simulink model "model_lqr_1D"  (R2016b)
settings: Solver=FixedStepAuto  StartTime=0.0  StopTime=15  FixedStep=0.001  RelTol=1e-3  EnableMultiTasking=on
InitFcn:
  | initCallback_model1D
values from neighbouring files (symbols this model uses):
  C_phi = 6.2e-3    (= 0.0062)    [initCallback_model1D.m]
  C_psi = 3.1176e-5    (= 3.1176e-05)    [initCallback_model1D.m]
  g = 9.81    [initCallback_model1D.m]
  I_GO = I_KO + I_RM + m_R * l_AB^2    (= 0.00355187)    [initCallback_model1D.m]
  I_RM = 1.1683e-4    (= 0.00011683)    [initCallback_model1D.m]
  l_AB = 0.084    [initCallback_model1D.m]
  l_AC = 0.087    [initCallback_model1D.m]
  m_K = 0.221    [initCallback_model1D.m]
  m_R = 0.09    [initCallback_model1D.m]
  phi_0 = degtorad(3)    [initCallback_model1D.m]
  phi__d_0 = 0    [initCallback_model1D.m]
  psi_0 = 0    [initCallback_model1D.m]
  psi__d_0 = 0    [initCallback_model1D.m]
  T_M_e = 5.5e-4    (= 0.00055)    [initCallback_model1D.m]
  T_M_m = 12.4e-3    (= 0.0124)    [initCallback_model1D.m]
settings Model: Creator=ich  LastModifiedBy=ich
settings SolverCC: AutoInsertRateTranBlk=on
settings OptimizationCC: LifeSpan=inf
settings DebuggingCC: SFUnexpectedBacktrackingDiag=warning  SFNoUnconditionalDefaultTransitionDiag=warning  SFExecutionAtInitializationDiag=none
settings GRTTargetCC: TargetLangStandard=C89/C90 (ANSI)  GeneratePreprocessorConditionals=Disable all
settings ConfigComp: CovMetricSettings=dw  CovHtmlReporting=on  CovSaveCumulativeToWorkspaceVar=on  CovSaveSingleToWorkspaceVar=on  CovExternalEMLEnable=off

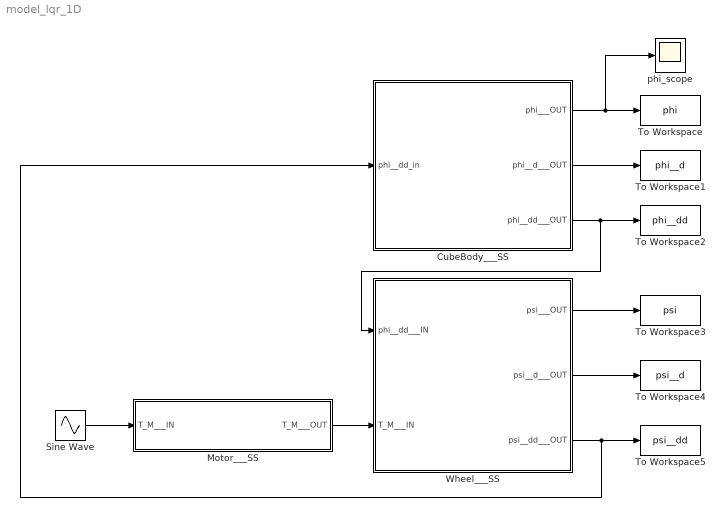
== system model_lqr_1D ==
  CubeBody___SS : Subsystem
  Motor___SS : Subsystem
  Sine Wave : Sin  Amplitude=0.05  SampleTime=0
  To Workspace : ToWorkspace  VariableName=phi  SaveFormat=Timeseries  SampleTime=-1
  To Workspace1 : ToWorkspace  VariableName=phi__d  SaveFormat=Timeseries  SampleTime=-1
  To Workspace2 : ToWorkspace  VariableName=phi__dd  SaveFormat=Timeseries  SampleTime=-1
  To Workspace3 : ToWorkspace  VariableName=psi  SaveFormat=Timeseries  SampleTime=-1
  To Workspace4 : ToWorkspace  VariableName=psi__d  SaveFormat=Timeseries  SampleTime=-1
  To Workspace5 : ToWorkspace  VariableName=psi__dd  SaveFormat=Timeseries  SampleTime=-1
  Wheel___SS : Subsystem
  phi_scope : Scope
  wires:
  Motor___SS/1(T_M___OUT) -> Wheel___SS/2(T_M___IN)
  CubeBody___SS/3(phi__dd___OUT) -> Wheel___SS/1(phi__dd___IN), To Workspace2/1
  Wheel___SS/3(psi__dd___OUT) -> To Workspace5/1, CubeBody___SS/1(phi__dd_in)
  CubeBody___SS/1(phi___OUT) -> phi_scope/1, To Workspace/1
  CubeBody___SS/2(phi__d___OUT) -> To Workspace1/1
  Wheel___SS/1(psi___OUT) -> To Workspace3/1
  Wheel___SS/2(psi__d___OUT) -> To Workspace4/1
  Sine Wave/1 -> Motor___SS/1(T_M___IN)

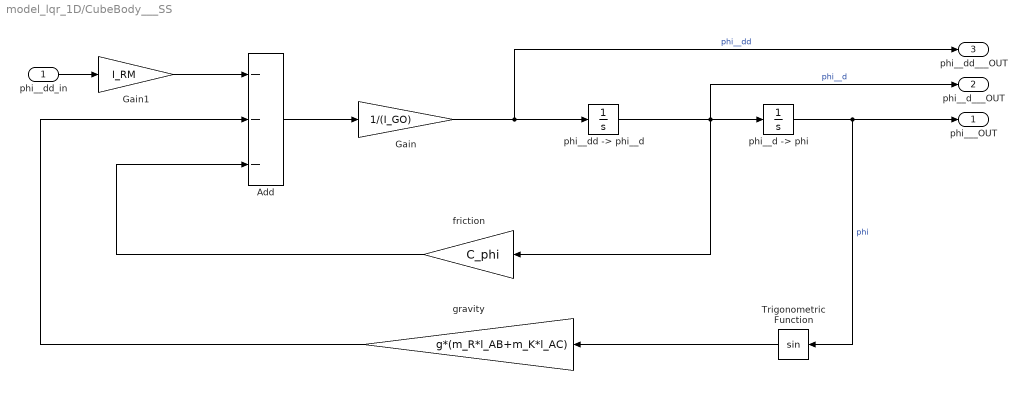
== system model_lqr_1D/CubeBody___SS ==
  phi__dd_in : Inport
  Add : Sum  Inputs=---
  Gain : Gain  Gain=1/(I_GO)
  Gain1 : Gain  Gain=I_RM
  Trigonometric Function : Trigonometry
  friction : Gain  Gain=C_phi
  gravity : Gain  Gain=g*(m_R*l_AB+m_K*l_AC)
  "phi__d -> phi" : Integrator  InitialCondition=phi_0
  "phi__dd -> phi__d" : Integrator  InitialCondition=phi__d_0
  phi___OUT : Outport
  phi__d___OUT : Outport  Port=2
  phi__dd___OUT : Outport  Port=3
  wires:
  "phi__d -> phi"/1 -> Trigonometric Function/1, phi___OUT/1  "phi"
  "phi__dd -> phi__d"/1 -> friction/1, phi__d___OUT/1, "phi__d -> phi"/1  "phi__d"
  Gain/1 -> phi__dd___OUT/1, "phi__dd -> phi__d"/1  "phi__dd"
  Add/1 -> Gain/1
  phi__dd_in/1 -> Gain1/1
  Gain1/1 -> Add/1
  Trigonometric Function/1 -> gravity/1
  gravity/1 -> Add/2
  friction/1 -> Add/3

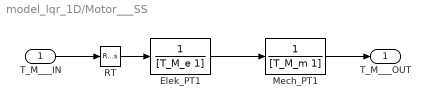
== system model_lqr_1D/Motor___SS ==
  T_M___IN : Inport
  Elek_PT1 : TransferFcn  Denominator=[T_M_e 1]
  Mech_PT1 : TransferFcn  Denominator=[T_M_m 1]
  RT : RateTransition  OutPortSampleTime=0.001
  T_M___OUT : Outport
  wires:
  T_M___IN/1 -> RT/1
  Elek_PT1/1 -> Mech_PT1/1
  Mech_PT1/1 -> T_M___OUT/1
  RT/1 -> Elek_PT1/1

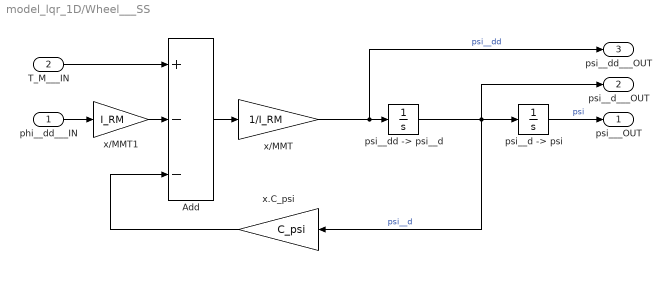
== system model_lqr_1D/Wheel___SS ==
  phi__dd___IN : Inport
  T_M___IN : Inport  Port=2
  Add : Sum  Inputs=+--
  "psi__d -> psi" : Integrator  InitialCondition=psi_0
  "psi__dd -> psi__d" : Integrator  InitialCondition=psi__d_0
  x.C_psi : Gain  Gain=C_psi
  x/MMT : Gain  Gain=1/I_RM
  x/MMT1 : Gain  Gain=I_RM
  psi___OUT : Outport
  psi__d___OUT : Outport  Port=2
  psi__dd___OUT : Outport  Port=3
  wires:
  "psi__d -> psi"/1 -> psi___OUT/1  "psi"
  "psi__dd -> psi__d"/1 -> psi__d___OUT/1, "psi__d -> psi"/1, x.C_psi/1  "psi__d"
  x/MMT/1 -> psi__dd___OUT/1, "psi__dd -> psi__d"/1  "psi__dd"
  Add/1 -> x/MMT/1
  T_M___IN/1 -> Add/1
  x.C_psi/1 -> Add/3
  phi__dd___IN/1 -> x/MMT1/1
  x/MMT1/1 -> Add/2
